simulink model "Overall_Schematic"  (R2016a)
settings: Solver=VariableStepAuto  StartTime=0.0  StopTime=20  RelTol=1e-3
libraries: powerlib x34
settings Model: Creator=DELL  LastModifiedBy=DELL

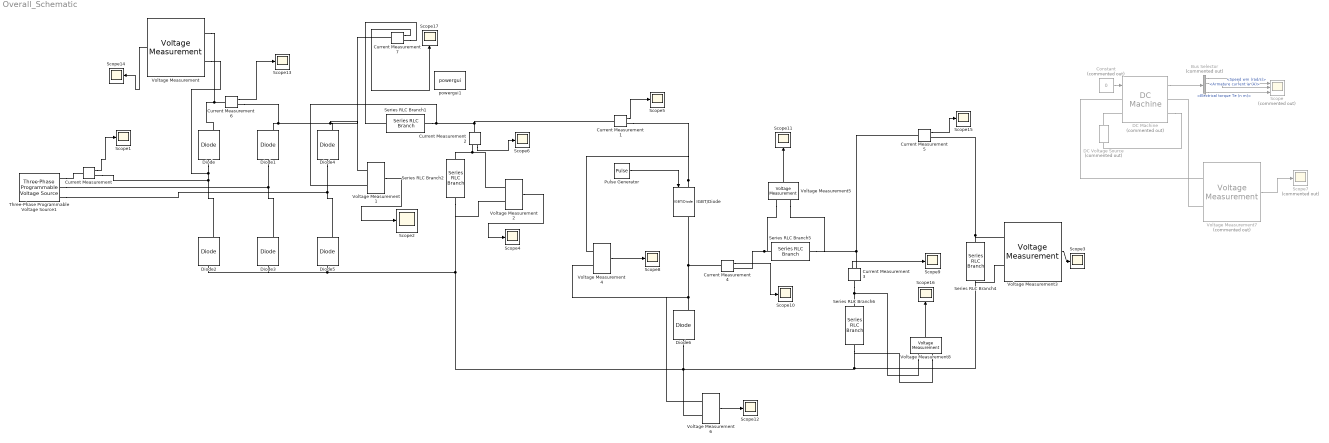
== system Overall_Schematic ==
  Bus Selector : BusSelector  Commented=on  OutputSignals=Speed wm (rad/s),Armature current ia (A),Field current if (A),Electrical torque Te (n m)
  Constant : Constant  Commented=on  Value=0
  Current Measurement{,1..7} (8 alike) : powerlib/Measurements/Current Measurement  PhasorSimulation=off  OutputType=Complex  PSBequivalent=0
  DC Machine : powerlib/Machines/DC Machine  Commented=on  PresetModel=No  MechanicalLoad=Torque TL  FieldType=Wound  ShowDetailedParameters=on  MeasurementBus=off  RLa="[ 28  0.0133]"  RLf="[ 8260  6.4]"  Laf=5  MachineConstant=Torque constant (N.m/A)  Ke=1.8  Kt=1.8  J=1  Bm=0  Tf=0  w0=0  Ifinit=1  TsPowergui=0  TsBlock=-1
  DC Voltage Source : powerlib/Electrical Sources/DC Voltage Source  Commented=on  Amplitude=300  Measurements=None
  Diode{,1..5} (6 alike) : powerlib/Power Electronics/Diode  Ron=0.02  Lon=0  Vf=0.8  IC=0  UseSnubber=off  Rs=500  Cs=250e-9  Measurements=on
  Diode6 : powerlib/Power Electronics/Diode  Ron=0.001  Lon=0  Vf=0.8  IC=0  UseSnubber=off  Rs=500  Cs=250e-9  Measurements=on
  IGBT/Diode : powerlib/Power Electronics/IGBT//Diode  Ron=1e-3  Rs=1e5  Cs=inf  Measurements=on
  Pulse Generator : DiscretePulseGenerator  PulseType=Time based  Period=1/10000  PulseWidth=80
  Scope : Scope  Commented=on  NumInputPorts=3
  Scope{1..6,8..17} (16 alike) : Scope
  Scope7 : Scope  Commented=on
  Series RLC Branch1 : powerlib/Elements/Series RLC Branch  LConnTagsString=__new0  RConnTagsString=__new0  BranchType=L  Resistance=30  Inductance=270e-6  SetiL0=off  InitialCurrent=0  Capacitance=1e-6  Setx0=off  InitialVoltage=0  Measurements=None
  Series RLC Branch2 : powerlib/Elements/Series RLC Branch  LConnTagsString=__new0  RConnTagsString=__new0  BranchType=C  Resistance=30  Inductance=13.3e-3  SetiL0=off  InitialCurrent=0  Capacitance=680e-6  Setx0=off  InitialVoltage=0  Measurements=None
  Series RLC Branch4 : powerlib/Elements/Series RLC Branch  LConnTagsString=__new0  RConnTagsString=__new0  BranchType=R  Resistance=55  Inductance=150e-3  SetiL0=off  InitialCurrent=0  Capacitance=1e-6  Setx0=off  InitialVoltage=0  Measurements=None
  Series RLC Branch5 : powerlib/Elements/Series RLC Branch  LConnTagsString=__new0  RConnTagsString=__new0  BranchType=L  Resistance=30  Inductance=270e-6  SetiL0=off  InitialCurrent=0  Capacitance=1e-6  Setx0=off  InitialVoltage=0  Measurements=None
  Series RLC Branch6 : powerlib/Elements/Series RLC Branch  LConnTagsString=__new0  RConnTagsString=__new0  BranchType=C  Resistance=30  Inductance=13.3e-3  SetiL0=off  InitialCurrent=0  Capacitance=680e-6  Setx0=off  InitialVoltage=0  Measurements=None
  Three-Phase Programmable Voltage Source1 : powerlib/Electrical Sources/Three-Phase Programmable Voltage Source  PositiveSequence="[95*sqrt(3)  0 50]"  VariationEntity=None  VariationType=Table of time-amplitude pairs  VariationTypeAlt=Step  VariationStep=0.5  VariationRate=10  VariationMagnitude=0.3  VariationFrequency=2  VariationTiming=[1 2]  VariationPhaseA=off  Amplitudes=[1 0.8 1.2 1.0]  TimeValues=[0 0.1 0.15 0.2]  HarmonicGeneration=off  HarmonicA=[3 0.2 -25 0]  HarmonicB=[2 0.15 35 2]  Timing="[0.05  3]"  BusType=swing  Pref=0  Qref=0  Qmin=-inf  Qmax=inf
  Voltage Measurement{,1..6,8} (8 alike) : powerlib/Measurements/Voltage Measurement  PhasorSimulation=off  OutputType=Complex  PSBequivalent=0
  Voltage Measurement7 : powerlib/Measurements/Voltage Measurement  Commented=on  PhasorSimulation=off  OutputType=Complex  PSBequivalent=0
  powergui1 : powerlib/powergui  Priority=1  SimulationMode=Discrete  SolverType=Tustin/Backward Euler (TBE)  SampleTime=1e-5  frequency=60  SPID=off  DisableSnubberDevices=off  DisableRonSwitches=off  DisableVfSwitches=off  SwTol=0  DisplayEquations=off  Interpol=off  ExternalGateDelay=off  methode=off  Ts=10  FunctionMessages=off  echomessages=off  HookPort=off  EnableUseOfTLC=off  x0status=blocks  frequencyindice=0  Pbase=100e6  ErrMax=1e-4  Iterations=50  UnitsV=kV  UnitsW=MW  buscounter=0  RestoreLinks=warning  ResistiveCurrentMeasurement=off  Frange=[0:2:500]  Ylog=off  Xlog=on  ShowGrid=off  save=off  variable=ZData  structure=0  ZoomFFT=off  StartTime=0.0  cycles=1  DisplayStyle=1  fundamental=60  FreqAxis=off  MaxFrequency=1000  frequencyindicesteady=1  RmsSteady=1  display=off
  wires:
  Current Measurement/1 -> Scope1/1
  Voltage Measurement2/1 -> Scope4/1
  Current Measurement1/1 -> Scope5/1
  Voltage Measurement1/1 -> Scope2/1
  Voltage Measurement3/1 -> Scope3/1
  Pulse Generator/1 -> IGBT/Diode/1
  Voltage Measurement4/1 -> Scope8/1
  Current Measurement3/1 -> Scope9/1
  Current Measurement4/1 -> Scope10/1
  Voltage Measurement5/1 -> Scope11/1
  Voltage Measurement6/1 -> Scope12/1
  Current Measurement5/1 -> Scope15/1
  Current Measurement2/1 -> Scope6/1
  Constant/1 -> DC Machine/1
  DC Machine/1 -> Bus Selector/1
  Bus Selector/1 -> Scope/1  "<Speed wm (rad/s)>"
  Bus Selector/2 -> Scope/2  "<Armature current ia (A)>"
  Bus Selector/4 -> Scope/3  "<Electrical torque Te (n m)>"
  Voltage Measurement7/1 -> Scope7/1
  Current Measurement6/1 -> Scope13/1
  Voltage Measurement/1 -> Scope14/1
  Voltage Measurement8/1 -> Scope16/1
  Current Measurement7/1 -> Scope17/1
  connections:
  Diode1/LConn1 -- Three-Phase Programmable Voltage Source1/RConn2 -- Diode3/RConn1
  Diode4/LConn1 -- Three-Phase Programmable Voltage Source1/RConn3 -- Diode5/RConn1
  Diode1/RConn1 -- Current Measurement6/RConn1 -- Current Measurement7/LConn1 -- Voltage Measurement1/LConn1 -- Diode4/RConn1
  Diode/LConn1 -- Voltage Measurement/LConn2 -- Current Measurement/RConn1 -- Diode2/RConn1
  Three-Phase Programmable Voltage Source1/RConn1 -- Current Measurement/LConn1
  Voltage Measurement2/LConn1 -- Series RLC Branch2/LConn1 -- Current Measurement2/RConn1
  Series RLC Branch1/LConn1 -- Voltage Measurement1/LConn2 -- Current Measurement1/LConn1 -- Current Measurement2/LConn1
  Current Measurement3/RConn1 -- Current Measurement5/LConn1 -- Series RLC Branch5/LConn1 -- Voltage Measurement5/LConn2
  IGBT/Diode/LConn1 -- Current Measurement1/RConn1 -- Voltage Measurement4/LConn1
  Voltage Measurement5/LConn1 -- Series RLC Branch5/RConn1 -- Current Measurement4/RConn1
  Current Measurement4/LConn1 -- IGBT/Diode/RConn1 -- Diode6/RConn1 -- Voltage Measurement6/LConn1 -- Voltage Measurement4/LConn2
  Current Measurement3/LConn1 -- Voltage Measurement8/LConn1 -- Series RLC Branch6/LConn1
  DC Machine/RConn2 -- DC Voltage Source/LConn1
  DC Voltage Source/RConn1 -- DC Machine/LConn2
  Voltage Measurement6/LConn2 -- Voltage Measurement8/LConn2 -- Series RLC Branch6/RConn1 -- Voltage Measurement3/LConn2 -- Series RLC Branch4/LConn1 -- Diode2/LConn1 -- Diode3/LConn1 -- Diode5/LConn1 -- Series RLC Branch2/RConn1 -- Voltage Measurement2/LConn2 -- Diode6/LConn1
  DC Machine/LConn1 -- Voltage Measurement7/LConn1
  Voltage Measurement7/LConn2 -- DC Machine/RConn1
  Series RLC Branch4/RConn1 -- Current Measurement5/RConn1 -- Voltage Measurement3/LConn1
  Diode/RConn1 -- Voltage Measurement/LConn1 -- Current Measurement6/LConn1
  Current Measurement7/RConn1 -- Series RLC Branch1/RConn1
